simulink model "LFRefMdl"  (R2020a)
settings: Solver=FixedStepDiscrete  StartTime=0.0  StopTime=inf  FixedStep=Ts  RelTol=1e-3
values from neighbouring files (symbols this model uses):
  posSelector = [1,0,0,0,0,0; 0,0,1,0,0,0]    [helperLFSetUp.m]
  PredictionHorizon = 30    [helperLFSetUp.m]
  time_gap = 1.5    [helperLFSetUp.m]
  Ts = 0.1    [helperLFSetUp.m]
libraries: drivinglib x2, mpcadaslib x1
settings Model: Creator=The MathWorks, Inc.  LastModifiedBy=NAGARJUN
settings DataIOCC: SaveOutput=off  SaveTime=off  ReturnWorkspaceOutputs=off
settings OptimizationCC: DefaultParameterBehavior=Inlined  DefaultUnderspecifiedDataType=single  EnhancedBackFolding=on  PassReuseOutputArgsAs=Individual arguments  ZeroExternalMemoryAtStartup=off  ZeroInternalMemoryAtStartup=off  OptimizeBlockOrder=speed  DifferentSizesBufferReuse=on  OptimizationCustomize=off  EfficientTunableParamExpr=on
settings DebuggingCC: ParameterPrecisionLossMsg=none  ParameterTunabilityLossMsg=error  PregeneratedLibrarySubsystemCodeDiagnostic=none  ArithmeticOperatorsInVariantConditions=warning
settings HardwareCC: ProdLongLongMode=on
settings SFSimCC: SimUseLocalCustomCode=off  MATLABDynamicMemAlloc=off  CustomCodeUndefinedFunction=UseInterfaceOnly
settings RTWCC: SystemTargetFile=ert.tlc  TemplateMakefile=ert_default_tmf  GenerateReport=on  RTWUseLocalCustomCode=off  BuildConfiguration=Faster Runs  IncludeHyperlinkInReport=on  LaunchReport=on  TargetLang=C++  GenerateTraceInfo=on  GenerateTraceReport=on  GenerateTraceReportSl=on  GenerateTraceReportSf=on  GenerateTraceReportEml=on
settings CodeAppCC: ForceParamTrailComments=on  IgnoreCustomStorageClasses=off  MaxIdLength=63  OperatorAnnotations=on  SimulinkDataObjDesc=on  SFDataObjDesc=on  CustomSymbolStrFcn=$N$M$F  InsertBlockDesc=on
settings ERTTargetCC: TargetLangStandard=C++03 (ISO)  GenerateSampleERTMain=on  MultiInstanceERTCode=on  CodeInterfacePackaging=C++ class  InlinedParameterPlacement=NonHierarchical  RootIOFormat=Structure reference  ERTCustomFileTemplate=example_file_process.tlc

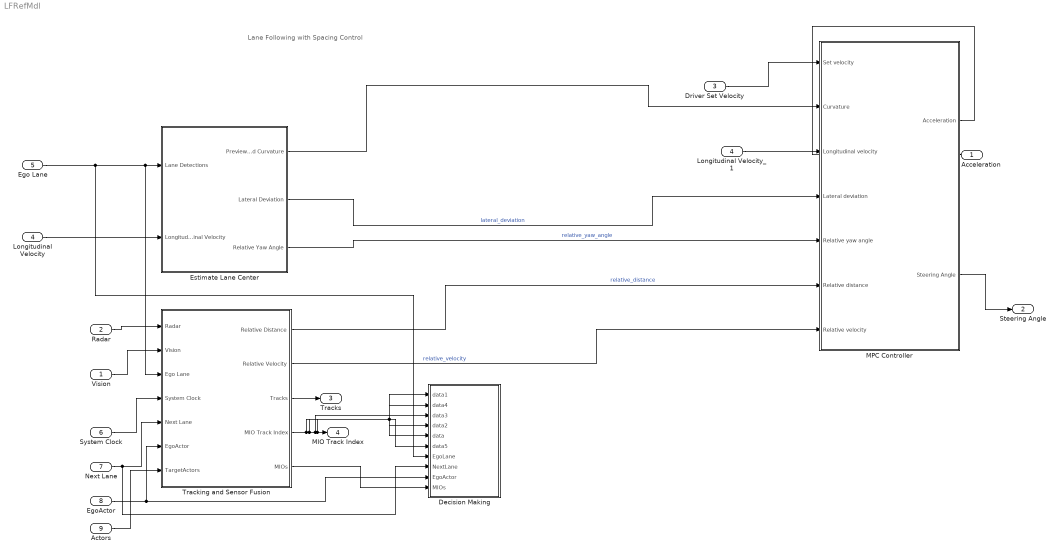
== system LFRefMdl ==
  note: Lane Following with Spacing Control
  Vision : Inport  OutDataTypeStr=Bus: BusVision  PortDimensions=[1 1]  BusOutputAsStruct=on
  Radar : Inport  Port=2  OutDataTypeStr=Bus: BusRadar  PortDimensions=[1 1]  BusOutputAsStruct=on
  Driver Set Velocity : Inport  Port=3
  Longitudinal Velocity : Inport  Port=4  OutDataTypeStr=double  Unit=m/s
  Ego Lane : Inport  Port=5  OutDataTypeStr=Bus: LaneSensor  PortDimensions=[1 1]
  System Clock : Inport  Port=6  OutDataTypeStr=double  PortDimensions=[1 1]
  Next Lane : Inport  Port=7  OutDataTypeStr=double  PortDimensions=[1 1]
  EgoActor : Inport  Port=8  OutDataTypeStr=double  PortDimensions=[1 1]
  Actors : Inport  Port=9  OutDataTypeStr=double  PortDimensions=[1 1]
  Decision Making : Stateflow chart  TreatAsAtomicUnit=on
  Estimate Lane Center : Subsystem  TreatAsAtomicUnit=on  VariantControl=v2
      settings: RTWFileNameOpts=Use function name
  Longitudinal Velocity_1 : InportShadow  Port=4  OutDataTypeStr=double  Unit=m/s
  "MPC Controller " : Subsystem
  Tracking and Sensor Fusion : Subsystem  TreatAsAtomicUnit=on
      settings: RTWFileNameOpts=Use function name
  Acceleration : Outport  PortDimensions=1  VectorParamsAs1DForOutWhenUnconnected=off
  Steering Angle : Outport  Port=2  PortDimensions=1  VectorParamsAs1DForOutWhenUnconnected=off
  Tracks : Outport  Port=3  OutDataTypeStr=Bus: BusMultiObjectTracker1  PortDimensions=[1 1]  VectorParamsAs1DForOutWhenUnconnected=off  BusOutputAsStruct=on
  MIO Track Index : Outport  Port=4  PortDimensions=1  VectorParamsAs1DForOutWhenUnconnected=off  BusOutputAsStruct=on
  wires:
  Longitudinal Velocity/1 -> Estimate Lane Center/2(Longitudinal Velocity)
  Vision/1 -> Tracking and Sensor Fusion/2(Vision)
  Radar/1 -> Tracking and Sensor Fusion/1(Radar)
  System Clock/1 -> Tracking and Sensor Fusion/4(System Clock)
  Tracking and Sensor Fusion/3(Tracks) -> Tracks/1
  Tracking and Sensor Fusion/4(MIO Track Index) -> Decision Making/5(data), Decision Making/2(data4), Decision Making/4(data2), Decision Making/6(data5), Decision Making/3(data3), Decision Making/1(data1), MIO Track Index/1
  Driver Set Velocity/1 -> "MPC Controller "/1(Set velocity)
  Longitudinal Velocity_1/1 -> "MPC Controller "/3(Longitudinal velocity)
  Estimate Lane Center/1(Previewed Curvature) -> "MPC Controller "/2(Curvature)
  "MPC Controller "/1(Acceleration) -> Acceleration/1
  "MPC Controller "/2(Steering Angle) -> Steering Angle/1
  Estimate Lane Center/2(Lateral Deviation) -> "MPC Controller "/4(Lateral deviation)  "lateral_deviation"
  Estimate Lane Center/3(Relative Yaw Angle) -> "MPC Controller "/5(Relative yaw angle)  "relative_yaw_angle"
  Tracking and Sensor Fusion/1(Relative Distance) -> "MPC Controller "/6(Relative distance)  "relative_distance"
  Tracking and Sensor Fusion/2(Relative Velocity) -> "MPC Controller "/7(Relative velocity)  "relative_velocity"
  Next Lane/1 -> Decision Making/8(NextLane), Tracking and Sensor Fusion/5(Next Lane)
  EgoActor/1 -> Decision Making/9(EgoActor), Tracking and Sensor Fusion/6(EgoActor)
  Actors/1 -> Tracking and Sensor Fusion/7(TargetActors)
  Ego Lane/1 -> Decision Making/7(EgoLane), Tracking and Sensor Fusion/3(Ego Lane), Estimate Lane Center/1(Lane Detections)
  Tracking and Sensor Fusion/5(MIOs) -> Decision Making/10(MIOs)

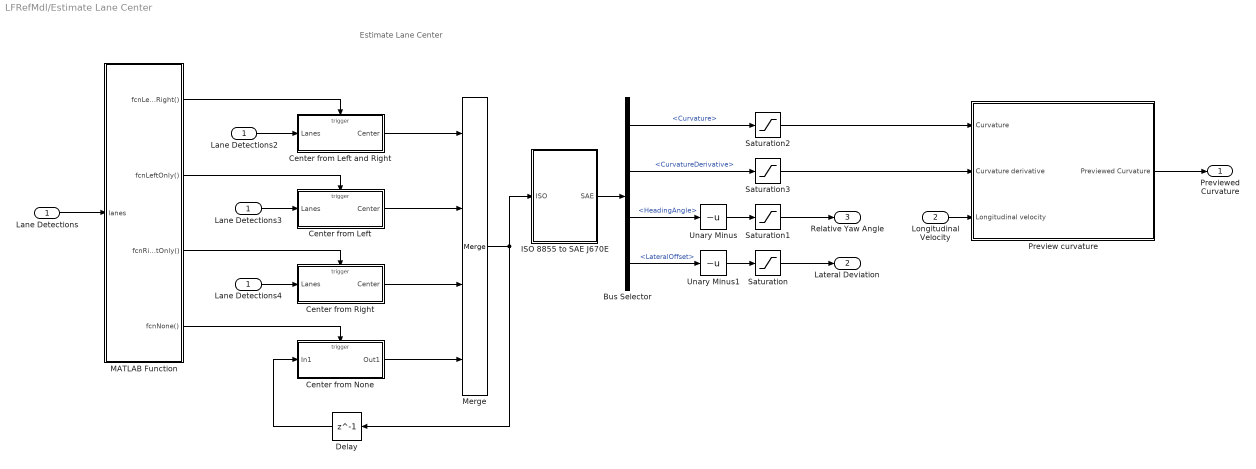
== system LFRefMdl/Estimate Lane Center ==
  note: Estimate Lane Center
  Lane Detections : Inport
  Longitudinal Velocity : Inport  Port=2
  Bus Selector : BusSelector  OutputSignals=Curvature,CurvatureDerivative,HeadingAngle,LateralOffset
  Center from Left : Subsystem  TreatAsAtomicUnit=on
  Center from Left and Right : Subsystem  TreatAsAtomicUnit=on
  Center from None : Subsystem  TreatAsAtomicUnit=on
  Center from Right : Subsystem  TreatAsAtomicUnit=on
  Delay : Delay  DelayLength=1
  ISO 8855 to SAE J670E : Subsystem
  Lane Detections2 : InportShadow
  Lane Detections3 : InportShadow
  Lane Detections4 : InportShadow
  MATLAB Function : MATLAB Function  TreatAsAtomicUnit=on
  Merge : Merge  Inputs=4
  Preview curvature : Subsystem
  Saturation : Saturate
  Saturation1 : Saturate  UpperLimit=0.6  LowerLimit=-0.6
  Saturation2 : Saturate  UpperLimit=0.15  LowerLimit=-0.15
  Saturation3 : Saturate  UpperLimit=0.06  LowerLimit=-0.06
  Unary Minus : UnaryMinus
  Unary Minus1 : UnaryMinus
  Previewed Curvature : Outport  VectorParamsAs1DForOutWhenUnconnected=off
  Lateral Deviation : Outport  Port=2  VectorParamsAs1DForOutWhenUnconnected=off
  Relative Yaw Angle : Outport  Port=3  VectorParamsAs1DForOutWhenUnconnected=off
  wires:
  Center from Right/1(Center) -> Merge/3
  Lane Detections3/1 -> Center from Left/1(Lanes)
  Lane Detections4/1 -> Center from Right/1(Lanes)
  MATLAB Function/2(fcnLeftOnly()) -> Center from Left/Trigger
  Center from None/1(Out1) -> Merge/4
  MATLAB Function/1(fcnLeftAndRight()) -> Center from Left and Right/Trigger
  Delay/1 -> Center from None/1(In1)
  Center from Left and Right/1(Center) -> Merge/1
  Lane Detections/1 -> MATLAB Function/1(lanes)
  Lane Detections2/1 -> Center from Left and Right/1(Lanes)
  MATLAB Function/3(fcnRightOnly()) -> Center from Right/Trigger
  MATLAB Function/4(fcnNone()) -> Center from None/Trigger
  Center from Left/1(Center) -> Merge/2
  Merge/1 -> ISO 8855 to SAE J670E/1(ISO), Delay/1
  Saturation3/1 -> Preview curvature/2(Curvature derivative)
  Saturation2/1 -> Preview curvature/1(Curvature)
  Saturation1/1 -> Relative Yaw Angle/1
  Saturation/1 -> Lateral Deviation/1
  Unary Minus/1 -> Saturation1/1
  Preview curvature/1(Previewed Curvature) -> Previewed Curvature/1
  Longitudinal Velocity/1 -> Preview curvature/3(Longitudinal velocity)
  Bus Selector/2 -> Saturation3/1  "<CurvatureDerivative>"
  Bus Selector/1 -> Saturation2/1  "<Curvature>"
  Unary Minus1/1 -> Saturation/1
  Bus Selector/4 -> Unary Minus1/1  "<LateralOffset>"
  Bus Selector/3 -> Unary Minus/1  "<HeadingAngle>"
  ISO 8855 to SAE J670E/1(SAE) -> Bus Selector/1

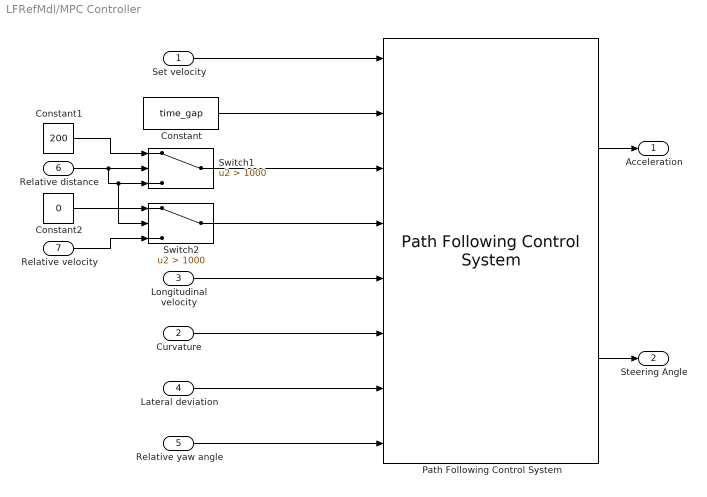
== system LFRefMdl/MPC Controller  ==
  Set velocity : Inport
  Curvature : Inport  Port=2
  Longitudinal velocity : Inport  Port=3
  Lateral deviation : Inport  Port=4
  Relative yaw angle : Inport  Port=5
  Relative distance : Inport  Port=6
  Relative velocity : Inport  Port=7
  Constant : Constant  Value=time_gap
  Constant1 : Constant  Value=200
  Constant2 : Constant  Value=0
  Path Following Control System : mpcadaslib/Path Following Control System  VariantControl=Variant2  ModelType=Use vehicle parameters  VehicleMass=m  VehicleYawInertia=Iz  LengthToFront=lf  LengthToRear=lr  FrontTireStiffness=Cf  RearTireStiffness=Cr  AccelTimeConstant=tau  EgoModelMatrixA=[-2,zeros(1,3);1,zeros(1,3);zeros(1,2),-4.4021,-12.4603;zeros(1,2),1.3913,-5.1868]  EgoModelMatrixB=[2,zeros(1,3);zeros(1,2),24.1270,15.8609]'  EgoModelMatrixC=[zeros(3,1),eye(3)]  InitialLongVel=v0_ego  TransportLag=Ts  spaceCtrl=on  DefaultSpacing=default_spacing  MinSteering=min_steer  umin_ext=off  MaxSteering=max_steer  umax_ext=off  MinAcceleration=min_ac  amin_ext=off  MaxAcceleration=max_ac  amax_ext=off  Ts=Ts  PredictionHorizon=PredictionHorizon  ControlHorizon=2  LongWeight=0.1  LateralWeight=1  AccelRateWeight=0.1  SteerRateWeight=0.1  suboptimal=off  maxiter=10  datatypeopt=double  optmode=off  trackmode=off
      settings: SourceProductBaseCode=MP
  Switch1 : Switch  Criteria=u2 > Threshold  Threshold=1000
  Switch2 : Switch  Criteria=u2 > Threshold  Threshold=1000
  Acceleration : Outport  VectorParamsAs1DForOutWhenUnconnected=off
  Steering Angle : Outport  Port=2  VectorParamsAs1DForOutWhenUnconnected=off
  wires:
  Path Following Control System/1 -> Acceleration/1
  Path Following Control System/2 -> Steering Angle/1
  Set velocity/1 -> Path Following Control System/1
  Curvature/1 -> Path Following Control System/6
  Longitudinal velocity/1 -> Path Following Control System/5
  Lateral deviation/1 -> Path Following Control System/7
  Relative yaw angle/1 -> Path Following Control System/8
  Constant/1 -> Path Following Control System/2
  Relative distance/1 -> Switch2/2, Switch1/3, Switch1/2
  Constant1/1 -> Switch1/1
  Switch1/1 -> Path Following Control System/3
  Relative velocity/1 -> Switch2/3
  Constant2/1 -> Switch2/1
  Switch2/1 -> Path Following Control System/4

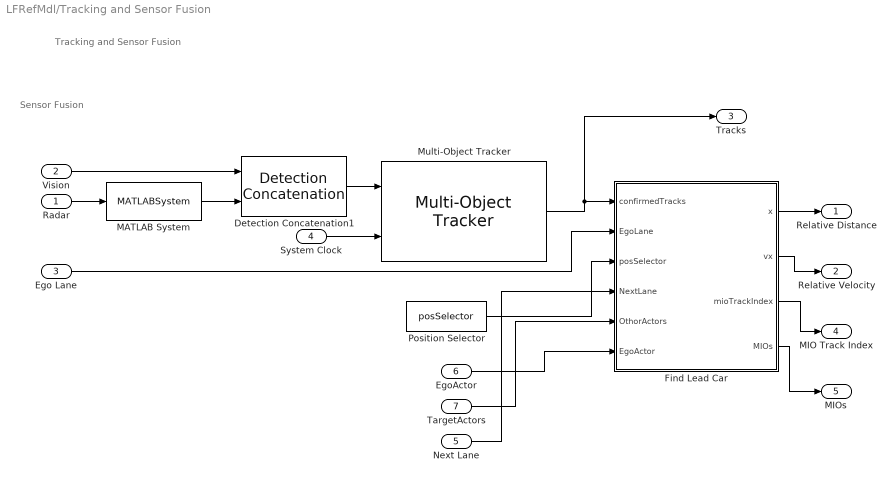
== system LFRefMdl/Tracking and Sensor Fusion ==
  note: Tracking and Sensor Fusion
  note: Sensor Fusion
  Radar : Inport  OutDataTypeStr=Bus: BusRadar  PortDimensions=[1 1]  BusOutputAsStruct=on
  Vision : Inport  Port=2  OutDataTypeStr=Bus: BusVision  PortDimensions=[1 1]  BusOutputAsStruct=on
  Ego Lane : Inport  Port=3  OutDataTypeStr=Bus: LaneSensor  BusOutputAsStruct=on
  System Clock : Inport  Port=4  OutDataTypeStr=double  PortDimensions=[1 1]
  Next Lane : Inport  Port=5  OutDataTypeStr=Bus: LaneSensor  BusOutputAsStruct=on
  EgoActor : Inport  Port=6  OutDataTypeStr=double  PortDimensions=[1 1]
  TargetActors : Inport  Port=7  OutDataTypeStr=double  PortDimensions=[1 1]
  Detection Concatenation1 : drivinglib/Detection Concatenation  NumInputs=2  BusNameSource=Auto  BusName=BusDetectionConcatenation1  SimulateUsing=Interpreted execution
      settings: SourceProductBaseCode=DR
  Find Lead Car : MATLAB Function  TreatAsAtomicUnit=on
  MATLAB System : MATLABSystem  System=helperClusterDetections  ClusterSize=clusterSize  BusNameSource=Auto  BusName=BusClusterDetections  SimulateUsing=Interpreted execution
      mask Type: helperClusterDetections
      mask Display:
      | disp(['Detection' char(10) 'Clustering']);
      | port_label('input',1,'In');
      | port_label('output',1,'Out');
  Multi-Object Tracker : drivinglib/Multi-Object Tracker  TrackerIndex=uint32( 0 )  FilterInitializationFcn=initcvekf  AssignmentThreshold=assigThresh  ConfirmationThreshold=[ 2, 3 ]  DeletionThreshold=[ 5, 5 ]  MaxNumTracks=numTracks  MaxNumSensors=numSensors  StateParams=struct  TimeInputSource=Input port  HasCostMatrixInput=off  HasDetectableTrackIDsInput=off  BusNameSource=Property  BusName=BusMultiObjectTracker1  TentativeTracksOutputPort=off  AllTracksOutputPort=off  SimulateUsing=Interpreted execution
      settings: SourceProductBaseCode=DR
  Position Selector : Constant  Value=posSelector
  Relative Distance : Outport  VectorParamsAs1DForOutWhenUnconnected=off
  Relative Velocity : Outport  Port=2  VectorParamsAs1DForOutWhenUnconnected=off
  Tracks : Outport  Port=3  OutDataTypeStr=Bus:BusMultiObjectTracker1  PortDimensions=[1 1]  VectorParamsAs1DForOutWhenUnconnected=off  BusOutputAsStruct=on
  MIO Track Index : Outport  Port=4  VectorParamsAs1DForOutWhenUnconnected=off
  MIOs : Outport  Port=5  VectorParamsAs1DForOutWhenUnconnected=off
  wires:
  Find Lead Car/2(vx) -> Relative Velocity/1
  Find Lead Car/3(mioTrackIndex) -> MIO Track Index/1
  Find Lead Car/1(x) -> Relative Distance/1
  Ego Lane/1 -> Find Lead Car/2(EgoLane)
  Detection Concatenation1/1 -> Multi-Object Tracker/1
  Multi-Object Tracker/1 -> Find Lead Car/1(confirmedTracks), Tracks/1
  Radar/1 -> MATLAB System/1
  System Clock/1 -> Multi-Object Tracker/2
  Vision/1 -> Detection Concatenation1/1
  MATLAB System/1 -> Detection Concatenation1/2
  Position Selector/1 -> Find Lead Car/3(posSelector)
  EgoActor/1 -> Find Lead Car/6(EgoActor)
  TargetActors/1 -> Find Lead Car/5(OthorActors)
  Next Lane/1 -> Find Lead Car/4(NextLane)
  Find Lead Car/4(MIOs) -> MIOs/1

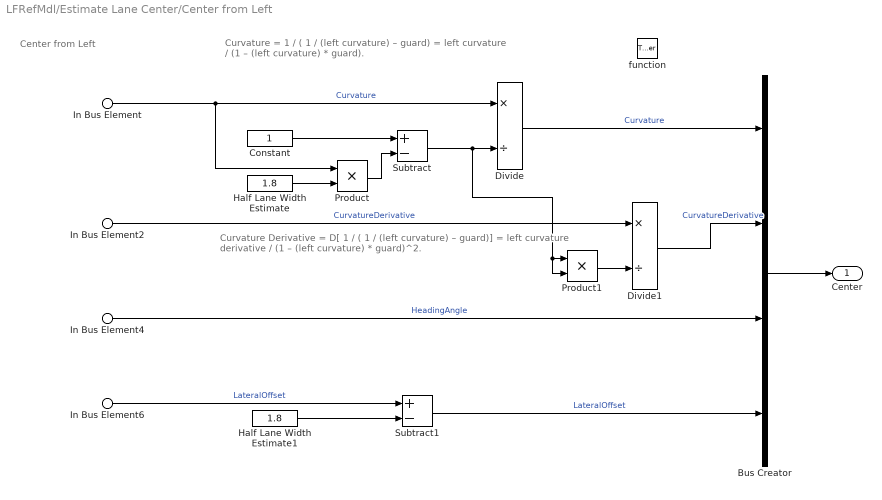
== system LFRefMdl/Estimate Lane Center/Center from Left ==
  note: Curvature Derivative
      | = D[ 1 / ( 1 / (left curvature) – guard)]
      | = left curvature derivative / (1 – (left curvature) * guard)^2.
  note: Center from Left
  note: Curvature
      | = 1 / ( 1 / (left curvature) – guard)
      | = left curvature / (1 – (left curvature) * guard).
  In Bus Element : Inport  PortName=Lanes  Element=Left.Curvature
  In Bus Element2 : Inport  PortName=Lanes  Element=Left.CurvatureDerivative
  In Bus Element4 : Inport  PortName=Lanes  Element=Left.HeadingAngle
  In Bus Element6 : Inport  PortName=Lanes  Element=Left.LateralOffset
  function : TriggerPort  TriggerType=function-call  VariantControl=Variant
  Bus Creator : BusCreator  Inputs=4
  Constant : Constant  OutDataTypeStr=Inherit: Inherit via back propagation
  Divide : Product  Inputs=*/
  Divide1 : Product  Inputs=*/
  Half Lane Width Estimate : Constant  Value=1.8  OutDataTypeStr=Inherit: Inherit via back propagation
  Half Lane Width Estimate1 : Constant  Value=1.8  OutDataTypeStr=Inherit: Inherit via back propagation
  Product : Product
  Product1 : Product
  Subtract : Sum  Inputs=+-
  Subtract1 : Sum  Inputs=+-
  Center : Outport  VectorParamsAs1DForOutWhenUnconnected=off
  wires:
  Product/1 -> Subtract/2
  Half Lane Width Estimate1/1 -> Subtract1/2
  In Bus Element6/1 -> Subtract1/1  "LateralOffset"
  Product1/1 -> Divide1/2
  In Bus Element2/1 -> Divide1/1  "CurvatureDerivative"
  Constant/1 -> Subtract/1
  Half Lane Width Estimate/1 -> Product/2
  Subtract/1 -> Divide/2, Product1/1, Product1/2
  In Bus Element/1 -> Divide/1, Product/1  "Curvature"
  Subtract1/1 -> Bus Creator/4  "LateralOffset"
  In Bus Element4/1 -> Bus Creator/3  "HeadingAngle"
  Divide/1 -> Bus Creator/1  "Curvature"
  Divide1/1 -> Bus Creator/2  "CurvatureDerivative"
  Bus Creator/1 -> Center/1

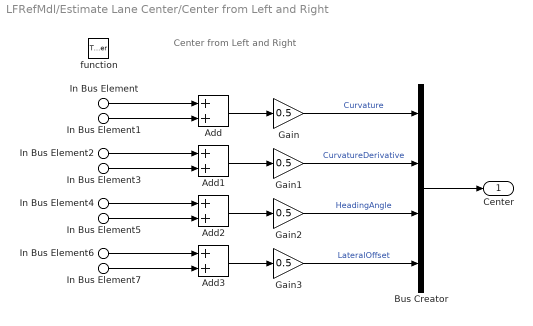
== system LFRefMdl/Estimate Lane Center/Center from Left and Right ==
  note: Center from Left and Right
  In Bus Element : Inport  PortName=Lanes  Element=Left.Curvature
  In Bus Element2 : Inport  PortName=Lanes  Element=Left.CurvatureDerivative
  In Bus Element4 : Inport  PortName=Lanes  Element=Left.HeadingAngle
  In Bus Element6 : Inport  PortName=Lanes  Element=Left.LateralOffset
  In Bus Element1 : Inport  PortName=Lanes  Element=Right.Curvature
  In Bus Element3 : Inport  PortName=Lanes  Element=Right.CurvatureDerivative
  In Bus Element5 : Inport  PortName=Lanes  Element=Right.HeadingAngle
  In Bus Element7 : Inport  PortName=Lanes  Element=Right.LateralOffset
  function : TriggerPort  TriggerType=function-call  VariantControl=Variant
  Add{,1..3} (4 alike) : Sum
  Bus Creator : BusCreator  Inputs=4
  Gain{,1..3} (4 alike) : Gain  Gain=0.5
  Center : Outport  VectorParamsAs1DForOutWhenUnconnected=off
  wires:
  In Bus Element6/1 -> Add3/1
  In Bus Element7/1 -> Add3/2
  In Bus Element5/1 -> Add2/2
  In Bus Element4/1 -> Add2/1
  In Bus Element3/1 -> Add1/2
  In Bus Element2/1 -> Add1/1
  In Bus Element1/1 -> Add/2
  In Bus Element/1 -> Add/1
  Bus Creator/1 -> Center/1
  Gain3/1 -> Bus Creator/4  "LateralOffset"
  Add3/1 -> Gain3/1
  Gain2/1 -> Bus Creator/3  "HeadingAngle"
  Add2/1 -> Gain2/1
  Gain1/1 -> Bus Creator/2  "CurvatureDerivative"
  Add1/1 -> Gain1/1
  Gain/1 -> Bus Creator/1  "Curvature"
  Add/1 -> Gain/1

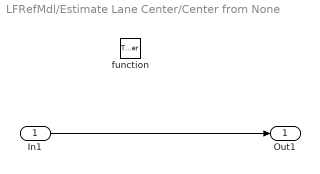
== system LFRefMdl/Estimate Lane Center/Center from None ==
  In1 : Inport
  function : TriggerPort  TriggerType=function-call  VariantControl=Variant
  Out1 : Outport  VectorParamsAs1DForOutWhenUnconnected=off
  wires:
  In1/1 -> Out1/1

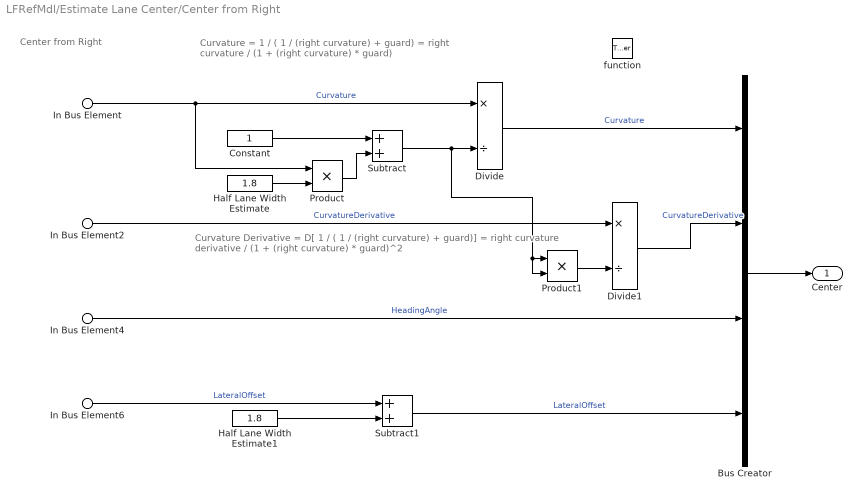
== system LFRefMdl/Estimate Lane Center/Center from Right ==
  note: Curvature Derivative
      | = D[ 1 / ( 1 / (right curvature) + guard)]
      | = right curvature derivative / (1 + (right curvature) * guard)^2
  note: Curvature
      | = 1 / ( 1 / (right curvature) + guard)
      | = right curvature / (1 + (right curvature) * guard)
  note: Center from Right
  In Bus Element : Inport  PortName=Lanes  Element=Right.Curvature
  In Bus Element2 : Inport  PortName=Lanes  Element=Right.CurvatureDerivative
  In Bus Element4 : Inport  PortName=Lanes  Element=Right.HeadingAngle
  In Bus Element6 : Inport  PortName=Lanes  Element=Right.LateralOffset
  function : TriggerPort  TriggerType=function-call  VariantControl=Variant
  Bus Creator : BusCreator  Inputs=4
  Constant : Constant  OutDataTypeStr=Inherit: Inherit via back propagation
  Divide : Product  Inputs=*/
  Divide1 : Product  Inputs=*/
  Half Lane Width Estimate : Constant  Value=1.8  OutDataTypeStr=Inherit: Inherit via back propagation
  Half Lane Width Estimate1 : Constant  Value=1.8  OutDataTypeStr=Inherit: Inherit via back propagation
  Product : Product
  Product1 : Product
  Subtract : Sum
  Subtract1 : Sum
  Center : Outport  VectorParamsAs1DForOutWhenUnconnected=off
  wires:
  Half Lane Width Estimate/1 -> Product/2
  Product/1 -> Subtract/2
  Constant/1 -> Subtract/1
  Subtract/1 -> Divide/2, Product1/1, Product1/2
  In Bus Element/1 -> Divide/1, Product/1  "Curvature"
  Bus Creator/1 -> Center/1
  Subtract1/1 -> Bus Creator/4  "LateralOffset"
  Divide/1 -> Bus Creator/1  "Curvature"
  In Bus Element6/1 -> Subtract1/1  "LateralOffset"
  Half Lane Width Estimate1/1 -> Subtract1/2
  In Bus Element4/1 -> Bus Creator/3  "HeadingAngle"
  Product1/1 -> Divide1/2
  Divide1/1 -> Bus Creator/2  "CurvatureDerivative"
  In Bus Element2/1 -> Divide1/1  "CurvatureDerivative"

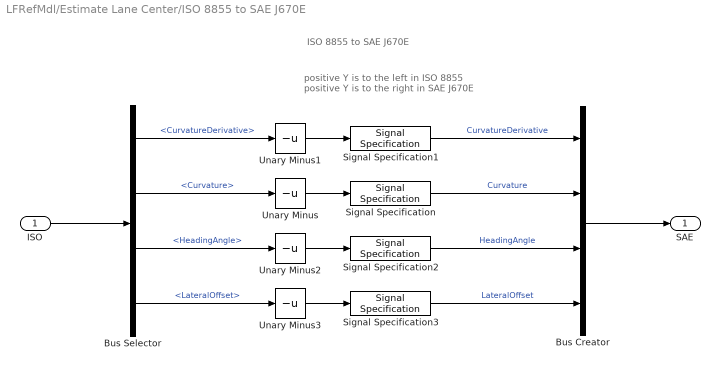
== system LFRefMdl/Estimate Lane Center/ISO 8855 to SAE J670E ==
  note: positive Y is to the left in ISO 8855
      | positive Y is to the right in SAE J670E
  note: ISO 8855 to SAE J670E
  ISO : Inport
  Bus Creator : BusCreator  Inputs=4
  Bus Selector : BusSelector  OutputSignals=CurvatureDerivative,Curvature,HeadingAngle,LateralOffset
  Signal Specification : SignalSpecification  Unit=1/m^2
  Signal Specification1 : SignalSpecification  Unit=1/m
  Signal Specification2 : SignalSpecification  Unit=rad
  Signal Specification3 : SignalSpecification  Unit=m
  Unary Minus{,1..3} (4 alike) : UnaryMinus
  SAE : Outport  VectorParamsAs1DForOutWhenUnconnected=off
  wires:
  ISO/1 -> Bus Selector/1
  Bus Selector/2 -> Unary Minus/1  "<Curvature>"
  Bus Selector/1 -> Unary Minus1/1  "<CurvatureDerivative>"
  Bus Selector/3 -> Unary Minus2/1  "<HeadingAngle>"
  Bus Selector/4 -> Unary Minus3/1  "<LateralOffset>"
  Bus Creator/1 -> SAE/1
  Signal Specification/1 -> Bus Creator/2  "Curvature"
  Unary Minus1/1 -> Signal Specification1/1
  Unary Minus2/1 -> Signal Specification2/1
  Unary Minus3/1 -> Signal Specification3/1
  Unary Minus/1 -> Signal Specification/1
  Signal Specification1/1 -> Bus Creator/1  "CurvatureDerivative"
  Signal Specification2/1 -> Bus Creator/3  "HeadingAngle"
  Signal Specification3/1 -> Bus Creator/4  "LateralOffset"

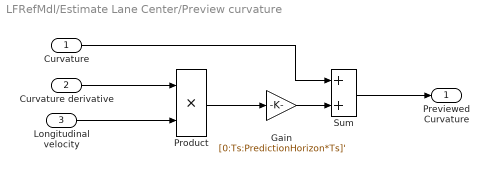
== system LFRefMdl/Estimate Lane Center/Preview curvature ==
  Curvature : Inport
  Curvature derivative : Inport  Port=2
  Longitudinal velocity : Inport  Port=3
  Gain : Gain  Gain=[0:Ts:PredictionHorizon*Ts]'
  Product : Product
  Sum : Sum
  Previewed Curvature : Outport  VectorParamsAs1DForOutWhenUnconnected=off
  wires:
  Sum/1 -> Previewed Curvature/1
  Curvature/1 -> Sum/1
  Gain/1 -> Sum/2
  Product/1 -> Gain/1
  Longitudinal velocity/1 -> Product/2
  Curvature derivative/1 -> Product/1

== matlab function LFRefMdl/Estimate Lane Center/MATLAB Function ==
  data: lanes input
  events: fcnLeftAndRight output FUNCTION_CALL_EVENT; fcnLeftOnly output FUNCTION_CALL_EVENT; fcnRightOnly output FUNCTION_CALL_EVENT; fcnNone output FUNCTION_CALL_EVENT
function fcn(lanes)

leftStrength  = lanes.Left.Strength;
rightStrength = lanes.Right.Strength;

if (leftStrength > 0) && (rightStrength > 0)
   fcnLeftAndRight();
   
elseif leftStrength > 0
    fcnLeftOnly();
    
elseif rightStrength > 0
    fcnRightOnly();
    
else
    fcnNone();
end

== stateflow chart LFRefMdl/Decision Making ==
  state Decision Logic
    state Lanefollwing
      {LFMode =true;
      %monitor the leading and follwing vehicle in ego lane
      {FCW.ZoneFront} = checkEgoFront();
      {FCW.ZoneRear} = checkEgoRear();
      %check if left Lane change is safe
      {SafeLF,SafeLR,ZoneLF,ZoneLR,LCParamLeft} =checkLCALeft();
      %check if Right Lane change is safe
      {SafeRF,SafeRR,ZoneRF,ZoneRR,LCParamLeft} =checkLCARight();
      }
      %Lane change to left
      {SafeLF &&SafeLR}
      {LCParam=LCParamLeft}
      %Lane change to Right
      {SafeRF &&SafeRR}
      {LCParam=LCParamRight}
      Lanefollwing -> (junction 16)
      (junction 24) -> (junction 18) : [duration(FCW) >0.6]
      (junction 16) -> (junction 19)
      (junction 18) -> (junction 21)
      (junction 21) -> (junction 22) [order 2]
      (junction 19) -> (junction 22)
    state LaneChange
      en:
      LCTrigger =true;
      LFMode =false;
      state StartDelay
      state CheckLCActive
        en:
        LCTrigger =false
        FCW =false;
      state WaitLCSettleDelay
      (default) -> StartDelay
      StartDelay -> CheckLCActive : {after(5,tick)}
      CheckLCActive -> WaitLCSettleDelay : [LCActive==false]
    LaneChange -> Lanefollwing : [after(LCSettleDelay, tick)]
    (junction 21) -> LaneChange [order 1]
    (junction 22) -> LaneChange
  (default) -> Lanefollwing
  data: data1 input; data4 input; data3 input; data2 input; data input; data5 input; EgoLane input; NextLane input; EgoActor input; MIOs input

== matlab function LFRefMdl/Tracking and Sensor Fusion/Find Lead Car ==
  data: confirmedTracks input; x output size=[1 1]; vx output size=[1 1]; EgoLane input; mioTrackIndex output; posSelector input; NextLane input; OthorActors input; EgoActor input; MIOs output
function [x,vx,mioTrackIndex,MIOs] = findLeadCar(confirmedTracks, EgoLane, posSelector,  NextLane, OthorActors, EgoActor)
% This function finds the lead car: a car in front of the ego car that
% satisfies all the criteria below:
% * Within the ego car's lane.
% * In front of the ego car.
% * Closest to the ego car.

% Note: If you change state definition, change the following:
%       State = [x;vx;y;vy;z;vz] (3D constant velocity)
numStates = 6;

% Initialize outputs and parameters
maxX = cast(1000, 'like', confirmedTracks.Tracks(1).State);  % Far enough forward so that no track is expected to exceed this distance
mioTrackIndex = 0;

% If lane detection is not available, the ego car is assumed to be located
% in the middle of its lane. The lane width is assumed to be 3.6m, typical
% highway lane width.
laneWidth = 3.6;
halfLaneWidth = laneWidth/2;

if EgoLane.Left.Strength > 0.01
    lb = [EgoLane.Left.CurvatureDerivative/6,...
        EgoLane.Left.Curvature/2,...
        EgoLane.Left.HeadingAngle,...
        EgoLane.Left.LateralOffset];
else
    lb = single([0,0,0,halfLaneWidth]);
end

if EgoLane.Right.Strength > 0.01
    rb = [EgoLane.Right.CurvatureDerivative/6,...
        EgoLane.Right.Curvature/2,...
        EgoLane.Right.HeadingAngle,...
        EgoLane.Right.LateralOffset];
else
    rb = single([0,0,0,-halfLaneWidth]);
end

% ego left lane detected?
if EgoLane.Left.Strength > 0.01 
    egoLeftLane = [EgoLane.Left.CurvatureDerivative/6,...
        EgoLane.Left.Curvature/2,...
        EgoLane.Left.HeadingAngle,...
        EgoLane.Left.LateralOffset];
else % ego left lane is not available
    egoLeftLane = single([0,0,0,halfLaneWidth]);
end
% ego right lane detected?
if EgoLane.Right.Strength > 0.01  
    egoRightLane = [EgoLane.Right.CurvatureDerivative/6,...
        EgoLane.Right.Curvature/2,...
        EgoLane.Right.HeadingAngle,...
        EgoLane.Right.LateralOffset];
else % ego right lane is not available
    egoRightLane = single([0,0,0,-halfLaneWidth]);    
end

% left next lane detected?
if NextLane.Left.Strength > 0.01 
    nextLeftLane = [NextLane.Left.CurvatureDerivative/6,...
        NextLane.Left.Curvature/2,...
        NextLane.Left.HeadingAngle,...
        NextLane.Left.LateralOffset];
else % left next lane is not available
    nextLeftLane = single([0,0,0,halfLaneWidth+laneWidth]);       
end
% right next lane detected?
if NextLane.Right.Strength > 0.01 
    nextRightLane = [NextLane.Right.CurvatureDerivative/6,...
        NextLane.Right.Curvature/2,...
        NextLane.Right.HeadingAngle,...
        NextLane.Right.LateralOffset];
else % right next lane is not available
    nextRightLane = single([0,0,0,halfLaneWidth+laneWidth]);       
end

% % Initialize outputs and parameters
% % Far enough forward so that no track is expected to exceed this distance
% egoMaxX = 500;
% % Far enough forward so that no track is expected to exceed this distance
% egoMinX = 500; %cast(-500, 'like', egoActor.Position);  
% % Far enough forward so that no track is expected to exceed this distance
% leftNextMaxX = 500;
% % Far enough rearward so that no track is expected to exceed this distance
% leftNextMinX = 500;
% % Far enough forward so that no track is expected to exceed this distance
% rightNextMaxX = 500;
% % Far enough rearward so that no track is expected to exceed this distance
% rightNextMinX = 500;

% Initialize outputs and parameters
% Far enough forward so that no track is expected to exceed this distance
egoMaxX = cast(500, 'like', EgoActor.Position);
% Far enough forward so that no track is expected to exceed this distance
egoMinX = cast(-500, 'like', EgoActor.Position);  
% Far enough forward so that no track is expected to exceed this distance
leftNextMaxX = cast(500, 'like', EgoActor.Position);  
% Far enough rearward so that no track is expected to exceed this distance
leftNextMinX = cast(-500, 'like', EgoActor.Position);  
% Far enough forward so that no track is expected to exceed this distance
rightNextMaxX = cast(500, 'like', EgoActor.Position); 
% Far enough rearward so that no track is expected to exceed this distance
rightNextMinX = cast(-500, 'like', EgoActor.Position);

% initialize MIOs
EgoFront = struct(...
    'TrackIndex', uint32(0),...
    'Position', double([0 0]'), ...
    'Velocity', double([0 0]'), ...
    'RangeMagnitude', double(2000), ...  % default range = big number (ex. 2000)
    'VelocityMagnitude', double(0), ...
    'TTC', double(100));

EgoRear = struct(...
    'TrackIndex', uint32(0),...
    'Position', double([0 0]'), ...
    'Velocity', double([0 0]'), ...
    'RangeMagnitude', double(0), ...  
    'VelocityMagnitude', double(0), ...
    'TTC', double(0));

LeftFront = struct(...
    'TrackIndex', uint32(0),...
    'Position', double([0 0]'), ...
    'Velocity', double([0 0]'), ...
    'RangeMagnitude', double(0), ...
    'VelocityMagnitude', double(0), ...
    'TTC', double(0));

LeftRear = struct(...
    'TrackIndex', uint32(0),...
    'Position', double([0 0]'), ...
    'Velocity', double([0 0]'), ...
    'RangeMagnitude', double(0), ...
    'VelocityMagnitude', double(0), ...
    'TTC', double(0));

RightFront = struct(...
    'TrackIndex', uint32(0),...
    'Position', double([0 0]'), ...
    'Velocity', double([0 0]'), ...
    'RangeMagnitude', double(0), ...
    'VelocityMagnitude', double(0), ...
    'TTC', double(0));

RightRear = struct(...
    'TrackIndex', uint32(0),...
    'Position', double([0 0]'), ...
    'Velocity', double([0 0]'), ...
    'RangeMagnitude', double(0), ...
    'VelocityMagnitude', double(0), ...
    'TTC', double(0));
MIOs = struct(...
    'NumMIOs',uint32(0),...
    'MIOObjects', repmat(RightFront,6,1));


for i = 1:confirmedTracks.NumTracks
    position = posSelector * confirmedTracks.Tracks(i).State;
    x = position(1); % Longitudinal position of the track relative to ego
    y = position(2); % Lateral position of the track relative to ego
    
    if x < maxX && x > 0 % No point checking otherwise

        yleftLane  = polyval(lb,x); % lateral position of left lane
        yrightLane = polyval(rb,x); % lateral position of right lane
        
        % Find a new lead car
        if (yrightLane <= y) && (y <= yleftLane)
            maxX = x;
            mioTrackIndex(:) = i;
        end
    end
end

if mioTrackIndex>0
    mioState = confirmedTracks.Tracks(mioTrackIndex).State;
else
    mioState = inf(numStates,1,'like',confirmedTracks.Tracks(1).State);
end

% Output:
x = mioState(1);    % Longitudinal position of the lead car
vx = mioState(2);   % Longitudinal velocity of the lead car

for i = 1:OthorActors.NumActors
    position = OthorActors.Actors(i).Position;
    % Longitudinal position of the target vehicle relative to ego
    x1 = position(1);
    % Lateral position of the target vehicle relative to ego
    y = position(2); 
    
    % lateral position of left ego lane   
    yEgoLaneLeft  = polyval(egoLeftLane,x1); 
     % lateral position of right ego lane
    yEgoLaneRight = polyval(egoRightLane,x1);
    
    % Check for ego front MIO
    if laneWidth < x1 && x1 < egoMaxX
        % Check for the target vehicles lane. Is it with in  the ego lane?
        if (yEgoLaneRight <= y) && (y <= yEgoLaneLeft) 
            egoMaxX = x1;
            % save track index for frontEgo MIO
            EgoFront.TrackIndex = uint32(i);
        end
    end   
    % Check of ego rear MIO
    if egoMinX < x1 && x1 < -1        
        if (yEgoLaneRight <= y) && (y <= yEgoLaneLeft)
            egoMinX = x1;
            % save track index for rearEgo MIO
            EgoRear.TrackIndex = uint32(i); 
        end
    end
    % Check for next lane
    if NextLane.Left.Strength > 0.01 
        % left next lane
        yNextLaneLeft = polyval(nextLeftLane,x1);  
        % right = ego left lane
        yNextLaneRight = polyval(egoLeftLane,x1); 
        
        % Check for left front MIO
        if 0 < x1 && x1 < leftNextMaxX            
            if (yNextLaneRight <= y) && (y <= yNextLaneLeft) 
                leftNextMaxX = x1;
                % save track index for nextFront MIO
                LeftFront.TrackIndex = uint32(i); 
            end
        end
        % Check for left rear MIO
        if leftNextMinX < x1 && x1 < 0            
            if (yNextLaneRight <= y) && (y <= yNextLaneLeft) 
                leftNextMinX = x1;
                % save track index for nextRear MIO
                LeftRear.TrackIndex = uint32(i); 
            end
        end
    end
    % left next lane detected?
    if NextLane.Right.Strength > 0.01 
        % left = ego right lane
        yNextLaneLeft = polyval(egoRightLane,x1); 
        % right next lane
        yNextLaneRight = polyval(nextRightLane,x1);  
        
        % Check for Ego right front MIO
        if 0 < x1 && x1 < rightNextMaxX            
            if (yNextLaneRight <= y) && (y <= yNextLaneLeft) 
                rightNextMaxX = x1;
                % save track index for nextFront MIO
                RightFront.TrackIndex = uint32(i); 
            end
        end
        % Check for Ego right rear MIO
        if rightNextMinX < x1 && x1 < 0            
            if (yNextLaneRight <= y) && (y <= yNextLaneLeft) 
                rightNextMinX = x1;
                % save track index for nextRear MIO
                RightRear.TrackIndex = uint32(i); 
            end
        end
    end    
end

% egoFront MIO detected?
if EgoFront.TrackIndex > 0 
    EgoFront.Position = OthorActors.Actors(EgoFront.TrackIndex).Position(1:2)';
    EgoFront.Velocity = OthorActors.Actors(EgoFront.TrackIndex).Velocity(1:2)';
    [EgoFront.RangeMagnitude, EgoFront.VelocityMagnitude, EgoFront.TTC] = ...
        calculateTTC(EgoFront.Position,EgoFront.Velocity);    
end
% egoRear MIO detected?
if EgoRear.TrackIndex > 0 
    EgoRear.Position = OthorActors.Actors(EgoRear.TrackIndex).Position(1:2)';
    EgoRear.Velocity = OthorActors.Actors(EgoRear.TrackIndex).Velocity(1:2)';
    [EgoRear.RangeMagnitude, EgoRear.VelocityMagnitude, EgoRear.TTC] = ...
        calculateTTC(EgoRear.Position,EgoRear.Velocity);    
end
% leftFront MIO detected?
if LeftFront.TrackIndex > 0 
    LeftFront.Position = OthorActors.Actors(LeftFront.TrackIndex).Position(1:2)';
    LeftFront.Velocity = OthorActors.Actors(LeftFront.TrackIndex).Velocity(1:2)';  
    [LeftFront.RangeMagnitude, LeftFront.VelocityMagnitude, LeftFront.TTC] = ...
        calculateTTC(LeftFront.Position,LeftFront.Velocity);    
end
% leftRear MIO detected? 
if LeftRear.TrackIndex > 0 
    LeftRear.Position = OthorActors.Actors(LeftRear.TrackIndex).Position(1:2)';
    LeftRear.Velocity = OthorActors.Actors(LeftRear.TrackIndex).Velocity(1:2)';    
    [LeftRear.RangeMagnitude, LeftRear.VelocityMagnitude, LeftRear.TTC] = ...
        calculateTTC(LeftRear.Position,LeftRear.Velocity);      
end
% dightFront MIO detected?
if RightFront.TrackIndex > 0 
    RightFront.Position = OthorActors.Actors(RightFront.TrackIndex).Position(1:2)';
    RightFront.Velocity = OthorActors.Actors(RightFront.TrackIndex).Velocity(1:2)';    
    [RightFront.RangeMagnitude, RightFront.VelocityMagnitude, RightFront.TTC] = ...
        calculateTTC(RightFront.Position,RightFront.Velocity);    
end
% rightRear MIO detected?
if RightRear.TrackIndex > 0  
    RightRear.Position = OthorActors.Actors(RightRear.TrackIndex).Position(1:2)';
    RightRear.Velocity = OthorActors.Actors(RightRear.TrackIndex).Velocity(1:2)';     
    [RightRear.RangeMagnitude, RightRear.VelocityMagnitude, RightRear.TTC] = ...
        calculateTTC(RightRear.Position,RightRear.Velocity);      
end
MIOs.NumMIOs = uint32(6);
MIOs.MIOObjects(1,1) = EgoFront;
MIOs.MIOObjects(2,1) = EgoRear;
MIOs.MIOObjects(3,1) = LeftFront;
MIOs.MIOObjects(4,1) = LeftRear;
MIOs.MIOObjects(5,1) = RightFront;
MIOs.MIOObjects(6,1) = RightRear;

end

% calculate magnitude of range and velocity, Time-to-contact (TTC) for MIO
function [RangeMagnitude,VelocityMagnitude,ttc] = calculateTTC(position,velocity)

[RangeAngle,RangeMagnitude] = cart2pol(position(1),position(2));
[VelocityAngle,vel] = cart2pol(velocity(1),velocity(2));

VelocityMagnitude = vel * cos(VelocityAngle-RangeAngle);
% limit speed to +/-0.1 m/s for ttc calculation
if abs(VelocityMagnitude)<0.1 
    if VelocityMagnitude>=0
        vel(:) = 0.1;
    else
        vel(:) = -0.1;
    end
else
    vel(:) = VelocityMagnitude;
end
% Time-To-Contact (sec)
ttc = RangeMagnitude/vel;
        
end
